simulink subsystem "Leds_esquiva"  (R2023b)
settings: Solver=VariableStepAuto  StartTime=0.0  StopTime=10.0  RelTol=1e-3
libraries: simulink x3
settings Model: Creator=alumnos  LastModifiedBy=Usuario_UMA

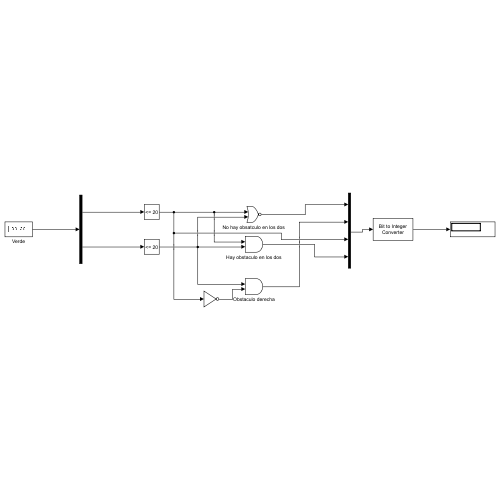
[thumbnail: Simulink's stored preview of the top-level diagram]
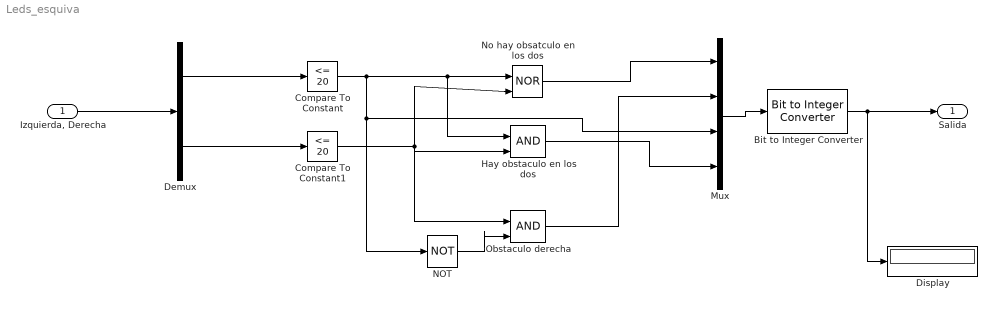
== system Leds_esquiva ==
  "Izquierda, Derecha" : Inport
  Bit to Integer Converter : simulink/Logic and Bit Operations/Bit to Integer Converter  nbits=4  bitOrder=MSB first  signedOutputValues=Unsigned  outDtype=Inherit via internal rule  outDtypeSigned=Inherit via internal rule
  Compare To Constant : simulink/Logic and Bit Operations/Compare To Constant  relop=<=  const=20  OutDataTypeStr=boolean
  Compare To Constant1 : simulink/Logic and Bit Operations/Compare To Constant  relop=<=  const=20  OutDataTypeStr=boolean
  Demux : Demux  Outputs=2
  Display : Display
  Hay obstaculo en los dos : Logic  IconShape=distinctive  AllPortsSameDT=off  OutDataTypeStr=boolean
  Mux : Mux
  NOT : Logic  Operator=NOT  IconShape=distinctive  AllPortsSameDT=off  OutDataTypeStr=boolean
  No hay obsatculo en los dos : Logic  Operator=NOR  IconShape=distinctive  AllPortsSameDT=off  OutDataTypeStr=boolean
  Obstaculo derecha : Logic  IconShape=distinctive  AllPortsSameDT=off  OutDataTypeStr=boolean
  Salida : Outport
  wires:
  "Izquierda, Derecha"/1 -> Demux/1
  Demux/1 -> Compare To Constant/1
  Demux/2 -> Compare To Constant1/1
  Compare To Constant/1 -> Mux/3, NOT/1, Hay obstaculo en los dos/1, No hay obsatculo en los dos/1
  Compare To Constant1/1 -> No hay obsatculo en los dos/2, Obstaculo derecha/1, Hay obstaculo en los dos/2
  NOT/1 -> Obstaculo derecha/2
  Mux/1 -> Bit to Integer Converter/1
  Bit to Integer Converter/1 -> Display/1, Salida/1
  No hay obsatculo en los dos/1 -> Mux/1
  Hay obstaculo en los dos/1 -> Mux/4
  Obstaculo derecha/1 -> Mux/2
